simulink model "modelsim"  (R2023b)
settings: Solver=VariableStepAuto  StartTime=0.0  StopTime=30.0  RelTol=1e-3
values from neighbouring files (symbols this model uses):
  A = [0 0 0 0 0 0 ... (first row only)    [rotation.m]
  B = [inv(J) ... (first row only)    [rotation.m]
  C = eye(6)    [rotation.m]
  D = zeros(6,3)    [rotation.m]
  G = transpose([0 0 0 0 0 0])    [rotation.m]
  I = transpose([omega, quat(2:4)])    [rotation.m]
undefined symbols (not defined in the file or in its folder): K, magnitude
libraries: aerolibconvert2 x1, sharedtransform x1
settings Model: Creator=satas  LastModifiedBy=jacksonwright

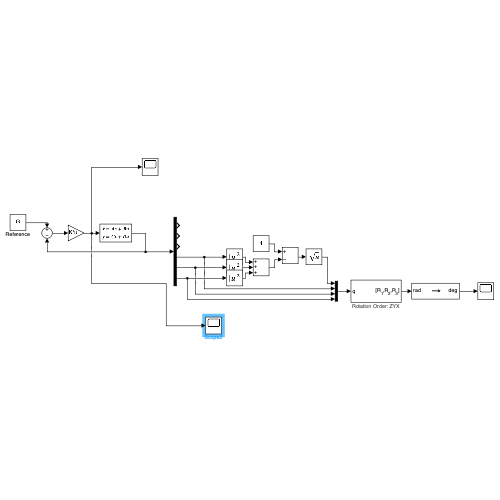
[thumbnail: Simulink's stored preview of the top-level diagram]
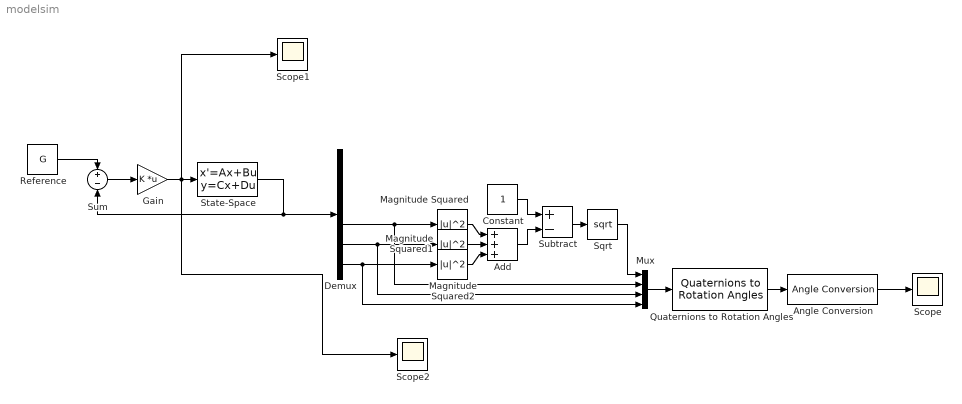
== system modelsim ==
  Add : Sum  Inputs=+++
  Angle Conversion : aerolibconvert2/Angle Conversion  IU=rad  OU=deg
  Constant : Constant
  Demux : Demux  Outputs=6
  Gain : Gain  Gain=K  Multiplication=Matrix(K*u)
  Magnitude Squared : Math  Operator=magnitude^2
  Magnitude Squared1 : Math  Operator=magnitude^2
  Magnitude Squared2 : Math  Operator=magnitude^2
  Mux : Mux
  Quaternions to Rotation Angles : sharedtransform/Quaternions to Rotation Angles  rotationOrder=ZYX  aMode=aMode
  Reference : Constant  Value=G
  Scope : Scope
  Scope1 : Scope
  Scope2 : Scope
  Sqrt : Sqrt
  State-Space : StateSpace  A=A  B=B  C=C  D=D  InitialCondition=I
  Subtract : Sum  Inputs=+-
  Sum : Sum  Inputs=+-
  wires:
  Reference/1 -> Sum/1
  State-Space/1 -> Demux/1, Sum/2
  Gain/1 -> Scope2/1, Scope1/1, State-Space/1
  Sum/1 -> Gain/1
  Demux/4 -> Mux/2, Magnitude Squared/1
  Demux/6 -> Mux/4, Magnitude Squared2/1
  Demux/5 -> Magnitude Squared1/1, Mux/3
  Mux/1 -> Quaternions to Rotation Angles/1
  Quaternions to Rotation Angles/1 -> Angle Conversion/1
  Constant/1 -> Subtract/1
  Magnitude Squared/1 -> Add/1
  Magnitude Squared1/1 -> Add/2
  Magnitude Squared2/1 -> Add/3
  Add/1 -> Subtract/2
  Subtract/1 -> Sqrt/1
  Sqrt/1 -> Mux/1
  Angle Conversion/1 -> Scope/1
